simulink model "serialrx"  (R2014b)
settings: Solver=ode45  StartTime=0.0  StopTime=inf  RelTol=1e-3
undefined symbols (not defined in the file): serial
libraries: instrumentlib x3
settings Model: Creator=Edoardo  LastModifiedBy=Edoardo

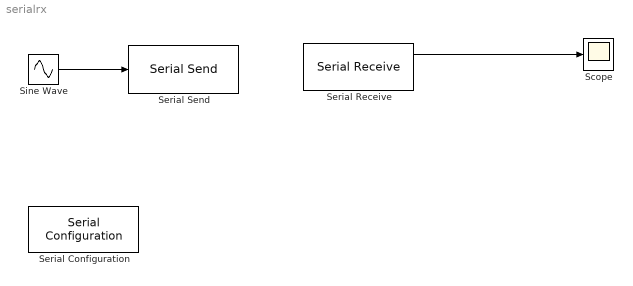
== system serialrx ==
  Scope : Scope
      settings: YMin=9  YMax=11.5
  Serial Configuration : instrumentlib/Serial Configuration  Priority=-200000  ComPortMenu=COM14  ComPort=COM14  ObjConstructor=serial('COM14');  BaudRate=115200  DataBits=8  Parity=none  StopBits=1  FlowControl=none  Timeout=10  ByteOrder=LittleEndian
  Serial Receive : instrumentlib/Serial Receive  ComPortMenu=COM14  ComPort=COM14  ObjConstructor=serial('COM14');  Terminator=<none>  DataSize=[1 1]  DataType=single  EnableBlockingMode=off  ActionDataUnavailable=Output last received value  CustomValue=0  SampleTime=0.01
  Serial Send : instrumentlib/Serial Send  ComPortMenu=COM14  ComPort=COM14  ObjConstructor=serial('COM14');  Terminator=<none>  EnableBlockingMode=off
  Sine Wave : Sin  SampleTime=0.1
  wires:
  Serial Receive/1 -> Scope/1
  Sine Wave/1 -> Serial Send/1
